simulink model "intro_2"  (R2025b)
settings: Solver=FixedStepAuto  StartTime=0.0  StopTime=10.0  FixedStep=1e-4  RelTol=1e-3
values from neighbouring files (symbols this model uses):
  a = 0.2    [setup.m]
  omega1 = 8    [setup.m]
  omega2 = 5    [setup.m]
  qbar1 = 1.5    [setup.m]
  qbar2 = 0.5    [setup.m]
settings Model: Creator=seby  LastModifiedBy=seby

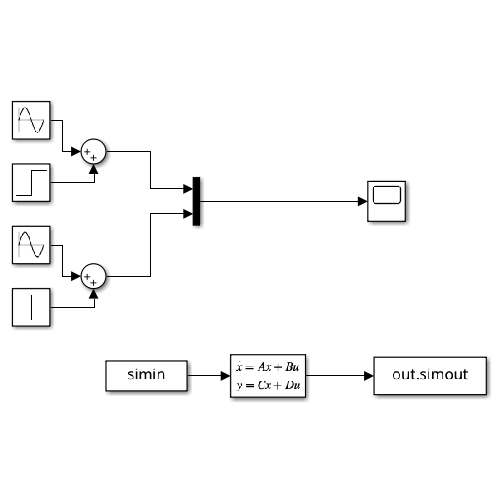
[thumbnail: Simulink's stored preview of the top-level diagram]
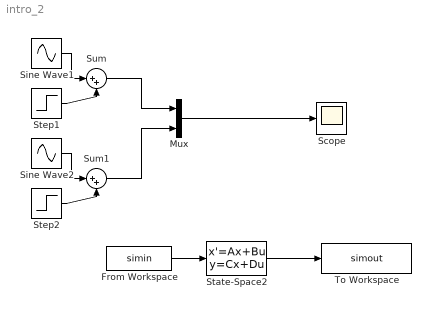
== system intro_2 ==
  From Workspace : FromWorkspace  VariableName=simin
  Mux : Mux  Inputs=2
  Scope : Scope
      settings: ActiveDisplayYMinimum=-1.8110529983174235  ActiveDisplayYMaximum=3.8333037218891466
  Sine Wave1 : Sin  Amplitude=a  Frequency=omega1  SampleTime=0
  Sine Wave2 : Sin  Amplitude=a  Frequency=omega2  SampleTime=0
  State-Space2 : StateSpace  A=[-3 0; 3 -5]  B=[1 0; 0 1]  C=[3 0; 0 5]  D=[0 0;0 0]  InitialCondition=[0.1;0.1]
  Step1 : Step  Time=0  After=qbar1  SampleTime=0
  Step2 : Step  Time=0  After=qbar2  SampleTime=0
  Sum : Sum  Inputs=|++
  Sum1 : Sum  Inputs=|++
  To Workspace : ToWorkspace  VariableName=simout  SaveFormat=Timeseries  SampleTime=-1
  wires:
  Mux/1 -> Scope/1
  Sine Wave1/1 -> Sum/1
  Step1/1 -> Sum/2
  Sine Wave2/1 -> Sum1/1
  Step2/1 -> Sum1/2
  Sum1/1 -> Mux/2
  Sum/1 -> Mux/1
  From Workspace/1 -> State-Space2/1
  State-Space2/1 -> To Workspace/1
